simulink model "Testecontrole"  (R2019b)
settings: Solver=FixedStepAuto  StartTime=0.0  StopTime=10.0  FixedStep=10^-3  RelTol=1e-3
values from neighbouring files (symbols this model uses):
  Ga1 = 1/7    (= 0.142857142857)    [varglobal.m]
  Gu1 = 1.8    [varglobal.m]
  Gv1 = 1/0.5    (= 2)    [varglobal.m]
  Gx1 = 1/0.5    (= 2)    [varglobal.m]
undefined symbols (not defined in the file or in its folder): K11
libraries: fuzblock x1
settings Model: Creator=aluno  LastModifiedBy=aluno

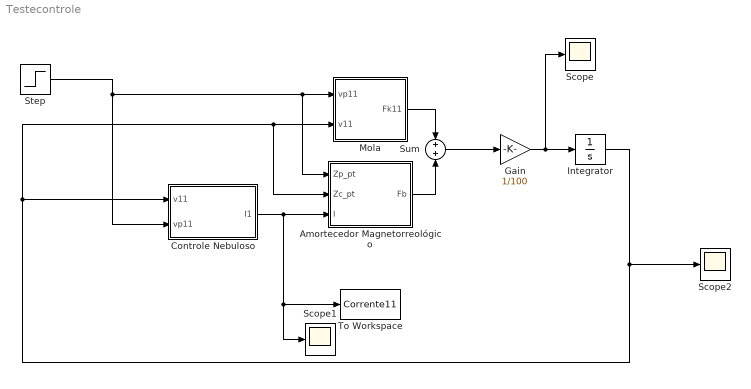
== system Testecontrole ==
  "Amortecedor Magnetorreológico " : Subsystem
  Controle Nebuloso : Subsystem
  Gain : Gain  Gain=1/100
  Integrator : Integrator
  Mola : Subsystem
  Scope : Scope
  Scope1 : Scope
  Scope2 : Scope
  Step : Step  Time=5  After=20  SampleTime=0
  Sum : Sum
  To Workspace : ToWorkspace  VariableName=Corrente11  SaveFormat=Timeseries  SampleTime=-1
  wires:
  Step/1 -> "Amortecedor Magnetorreológico "/1("Zp_pt "), Mola/1(vp11), Controle Nebuloso/2(vp11)
  Mola/1(Fk11) -> Sum/1
  Controle Nebuloso/1(I1) -> Scope1/1, To Workspace/1, "Amortecedor Magnetorreológico "/3(I)
  "Amortecedor Magnetorreológico "/1(Fb) -> Sum/2
  Integrator/1 -> Controle Nebuloso/1(v11), "Amortecedor Magnetorreológico "/2("Zc_pt "), Mola/2(v11), Scope2/1
  Sum/1 -> Gain/1
  Gain/1 -> Scope/1, Integrator/1

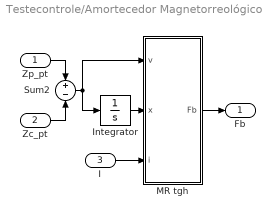
== system Testecontrole/Amortecedor Magnetorreológico  ==
  "Zp_pt " : Inport
  "Zc_pt " : Inport  Port=2
  I : Inport  Port=3
  Integrator : Integrator
  MR tgh : MATLAB Function  TreatAsAtomicUnit=on
  Sum2 : Sum  Inputs=+-
  Fb : Outport  VectorParamsAs1DForOutWhenUnconnected=off
  wires:
  MR tgh/1(Fb) -> Fb/1
  Integrator/1 -> MR tgh/2(x)
  "Zp_pt "/1 -> Sum2/1
  "Zc_pt "/1 -> Sum2/2
  I/1 -> MR tgh/3(i)
  Sum2/1 -> Integrator/1, MR tgh/1(v)

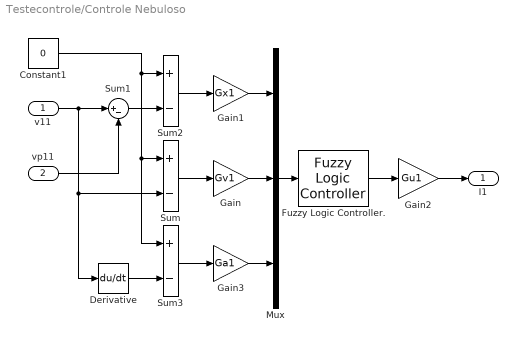
== system Testecontrole/Controle Nebuloso ==
  v11 : Inport
  vp11 : Inport  Port=2
  Constant1 : Constant  Value=0
  Derivative : Derivative
  Fuzzy Logic Controller. : fuzblock/Fuzzy Logic  Controller  FIS='Fuzzy_Sugeno.fis'  OutputSampleNumber=101  DataType=double  FuzzifiedInputs=off  RuleFiringStrengths=off  RuleOutputs=off  AggregatedOutputs=off  SimulateUsing=Interpreted execution  OutOfRangeInputValueMessage=warning  NoRuleFiredMessage=warning  EmptyOutputFuzzySetMessage=warning
  Gain : Gain  Gain=Gv1
  Gain1 : Gain  Gain=Gx1
  Gain2 : Gain  Gain=Gu1
  Gain3 : Gain  Gain=Ga1
  Mux : Mux  Inputs=3
  Sum : Sum  Inputs=+-
  Sum1 : Sum  Inputs=|+-
  Sum2 : Sum  Inputs=+-
  Sum3 : Sum  Inputs=+-
  I1 : Outport  VectorParamsAs1DForOutWhenUnconnected=off
  wires:
  Constant1/1 -> Sum3/1, Sum/1, Sum2/1
  Sum/1 -> Gain/1
  Sum2/1 -> Gain1/1
  Gain1/1 -> Mux/1
  Gain/1 -> Mux/2
  v11/1 -> Derivative/1, Sum/2, Sum1/1
  Gain3/1 -> Mux/3
  Sum3/1 -> Gain3/1
  Derivative/1 -> Sum3/2
  Gain2/1 -> I1/1
  Fuzzy Logic Controller./1 -> Gain2/1
  Mux/1 -> Fuzzy Logic Controller./1
  vp11/1 -> Sum1/2
  Sum1/1 -> Sum2/2

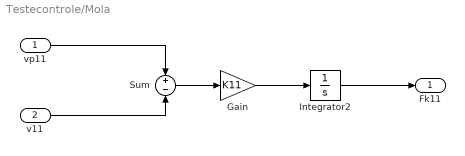
== system Testecontrole/Mola ==
  vp11 : Inport
  v11 : Inport  Port=2
  Gain : Gain  Gain=K11
  Integrator2 : Integrator
  Sum : Sum  Inputs=+-
  Fk11 : Outport  VectorParamsAs1DForOutWhenUnconnected=off
  wires:
  Sum/1 -> Gain/1
  Integrator2/1 -> Fk11/1
  v11/1 -> Sum/2
  vp11/1 -> Sum/1
  Gain/1 -> Integrator2/1

== matlab function Testecontrole/Amortecedor Magnetorreológico /MR tgh ==
  data: v input; x input; Fb output; i input
function Fb = tgh_model(v,x,i)
c = 9929*i+33340;
k = 0;
alpha = -144*i^2+5418*i+32;
beta = 100;
gamma = 0;
f0 = 0;
p = 1;
% p = 50;
% Fb = p*(k*x+c*v+alpha*tanh(beta*v+gamma*sign(x))+f0);
Fb = c*v+alpha*tanh(beta*v);
